simulink model "stable"  (R2020b)
settings: Solver=VariableStepAuto  StartTime=0.0  StopTime=40  RelTol=1e-3
undefined symbols (not defined in the file): c_1, c_2, g, Jp, Jr, L, Lp, Lr, Mp, x0
settings Model: Creator=5470  LastModifiedBy=5470

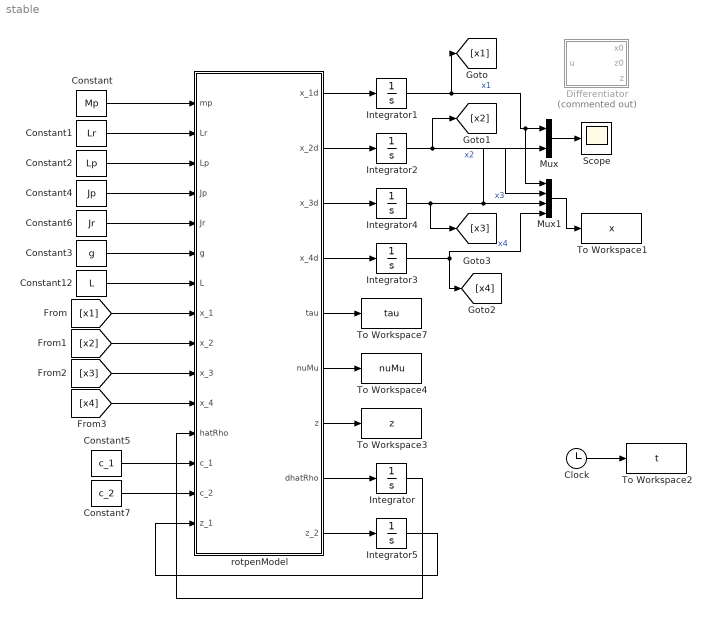
== system stable ==
  Clock : Clock
  Constant : Constant  Value=Mp
  Constant1 : Constant  Value=Lr
  Constant12 : Constant  Value=L
  Constant2 : Constant  Value=Lp
  Constant3 : Constant  Value=g
  Constant4 : Constant  Value=Jp
  Constant5 : Constant  Value=c_1
  Constant6 : Constant  Value=Jr
  Constant7 : Constant  Value=c_2
  Differentiator : Subsystem  Commented=on  TreatAsAtomicUnit=on  mask{n=1, r=3, Ts=-1, filtering=on, nf=1, differentiator_type=Set Homogeneity Degree manually, d=-1, m=1, mu=1}
      mask prompts: n "n ="; r "r ="; Ts "Ts ="; filtering "Enable Filtering"; nf "nf ="; differentiator_type "Type of Differentiator"; d "d ="; m "m ="; mu "mu ="
      mask Callback filtering:
      | zzzzzzzzzz_maskObj = Simulink.Mask.get(gcb);
      | 
      | zzzzzzzzzz_enabled = get_param(gcb, 'filtering');
      | 
      | zzzzzzzzzz_nf_group = zzzzzzzzzz_maskObj.getDialogControl('nf_group');
      | zzzzzzzzzz_nf_group.DialogControls(3).Visible = zzzzzzzzzz_enabled;
      | zzzzzzzzzz_maskVisibilities = get_param(gcb,'maskVisibilities');
      | zzzzzzzzzz_maskVisibilities{5} = zzzzzzzzzz_enabled;
      | set_param(gcb,'maskVisibilities', zzzzzzzzzz_maskVisibilities);
      | if(strcmp(zzzzzzzzzz_enabled, 'off') == 1)
      |     set_param(gcb, 'nf', '0');
      | end
      | 
      | clear zzzzzzzzzz_nf_group zzzzzzzzzz_enabled zzzzzzzzzz_maskVisibilities zzzzzzzzzz_maskObj;
      mask TypeOptions differentiator_type: Linear Differentiator | Robust Exact Differentiator | Uniform Robust Exact Differentiator | Set Homogeneity Degree manually
      mask Callback differentiator_type:
      | zzzzzzzzzz_maskObj = Simulink.Mask.get(gcb);
      | 
      | zzzzzzzzzz_diff_type = get_param(gcb, 'differentiator_type');
      | zzzzzzzzzz_enabled_m = 'on';
      | zzzzzzzzzz_enabled = 'on';
      | zzzzzzzzzz_enabled_m2 = 'off';
      | zzzzzzzzzz_enabled_m3 = 'off';
      | 
      | zzzzzzzzzz_val_m = str2double(get_param(gcb, 'm'));
      | 
      | if(strcmp(zzzzzzzzzz_diff_type, 'Set Homogeneity Degree manually') == 1)
      |     zzzzzzzzzz_enabled_m3 = 'on';
      | else
      |     zzzzzzzzzz_enabled = 'off';
      |     if(strcmp(zzzzzzzzzz_diff_type, 'Linear Differentiator') == 1)
      |         set_param(gcb, 'd', '0');
      |         if(zzzzzzzzzz_val_m == 2)
      |             set_param(gcb, 'm', '1');
      |         end
      |     elseif(strcmp(zzzzzzzzzz_diff_type, 'Robust Exact Differentiator') == 1)
      |         zzzzzzzzzz_enabled_m2 = 'on';
      | 
      |         set_param(gcb, 'd', '-1');
      |     elseif(strcmp(zzzzzzzzzz_diff_type, 'Uniform Robust Exact Differentiator') == 1)
      |         set_param(gcb, 'd', '-1');
      |         set_param(gcb, 'm', '2');
      | 
      |         zzzzzzzzzz_enabled_m = 'off';
      |     end
      | end
      | 
      | zzzzzzzzzz_d_group = zzzzzzzzzz_maskObj.getDialogControl('d_group');
      | zzzzzzzzzz_d_group.DialogControls(2).Visible = zzzzzzzzzz_enabled;
      | zzzzzzzzzz_maskVisibilities = get_param(gcb,'maskVisibilities');
      | zzzzzzzzzz_maskVisibilities{7} = zzzzzzzzzz_enabled;
      | 
      | zzzzzzzzzz_m_group = zzzzzzzzzz_maskObj.getDialogControl('m_group');
      | zzzzzzzzzz_m_group.Visible = zzzzzzzzzz_enabled_m;
      | zzzzzzzzzz_m_group.DialogControls(2).Visible = zzzzzzzzzz_enabled_m2;
      | zzzzzzzzzz_m_group.DialogControls(3).Visible = zzzzzzzzzz_enabled_m3;
      | set_param(gcb,'maskVisibilities', zzzzzzzzzz_maskVisibilities);
      | 
      | clear zzzzzzzzzz_d_group zzzzzzzzzz_maskVisibilities zzzzzzzzzz_m_group zzzzzzzzzz_enabled_m;
      | clear zzzzzzzzzz_enabled_m2 zzzzzzzzzz_enabled_m3 zzzzzzzzzz_enabled zzzzzzzzzz_diff_type;
      | clear zzzzzzzzzz_val_m;
      | 
      | 
      | 
      | zzzzzzzzzz_val_m = str2double(get_param(gcb, 'm'));
      | zzzzzzzzzz_val_d = str2double(get_param(gcb, 'd'));
      | zzzzzzzzzz_enabled_mu = 'off';
      | if((isnan(zzzzzzzzzz_val_m) || zzzzzzzzzz_val_m == 2) && (isnan(zzzzzzzzzz_val_d) || zzzzzzzzzz_val_d == -1))
      |     zzzzzzzzzz_enabled_mu = 'on';
      | end
      | zzzzzzzzzz_maskObj.getDialogControl('mu_group').Visible = zzzzzzzzzz_enabled_mu;
      | clear zzzzzzzzzz_val_m zzzzzzzzzz_val_d zzzzzzzzzz_enabled_mu zzzzzzzzzz_maskObj;
      | clear zzzzzzzzzz_maskObj
      mask Callback d:
      | zzzzzzzzzz_maskObj = Simulink.Mask.get(gcb);
      | zzzzzzzzzz_val_m = str2double(get_param(gcb, 'm'));
      | zzzzzzzzzz_val_d = str2double(get_param(gcb, 'd'));
      | zzzzzzzzzz_enabled_mu = 'off';
      | if((isnan(zzzzzzzzzz_val_m) || zzzzzzzzzz_val_m == 2) && (isnan(zzzzzzzzzz_val_d) || zzzzzzzzzz_val_d == -1))
      |     zzzzzzzzzz_enabled_mu = 'on';
      | end
      | zzzzzzzzzz_maskObj.getDialogControl('mu_group').Visible = zzzzzzzzzz_enabled_mu;
      | clear zzzzzzzzzz_val_m zzzzzzzzzz_val_d zzzzzzzzzz_enabled_mu zzzzzzzzzz_maskObj;
      | clear zzzzzzzzzz_maskObj
      mask Callback m:
      | zzzzzzzzzz_maskObj = Simulink.Mask.get(gcb);
      | zzzzzzzzzz_val_m = str2double(get_param(gcb, 'm'));
      | zzzzzzzzzz_val_d = str2double(get_param(gcb, 'd'));
      | zzzzzzzzzz_enabled_mu = 'off';
      | if((isnan(zzzzzzzzzz_val_m) || zzzzzzzzzz_val_m == 2) && (isnan(zzzzzzzzzz_val_d) || zzzzzzzzzz_val_d == -1))
      |     zzzzzzzzzz_enabled_mu = 'on';
      | end
      | zzzzzzzzzz_maskObj.getDialogControl('mu_group').Visible = zzzzzzzzzz_enabled_mu;
      | clear zzzzzzzzzz_val_m zzzzzzzzzz_val_d zzzzzzzzzz_enabled_mu zzzzzzzzzz_maskObj;
      | clear zzzzzzzzzz_maskObj
      mask DialogControl DescGroupVar Prompt: Differentiator Toolbox v3
      mask DialogControl DescTextVar Prompt: This block provides estimates of the derivatives of the input signal.
      mask DialogControl DescTextVar_2 Prompt: The first scalar output x0 provides a convergence measure. Increase the robustness factor 'r' to ensure that this signal converges to a sufficiently small neighborhood of zero.
      mask DialogControl DescTextVar_3 Prompt: The second output z0 is an estimate of the input signal.
      mask DialogControl DescTextVar_4 Prompt: The third output z is a vector containing the estimated derivatives of the input signal. The length of this vector equals the chosen differentiaton order 'n'.
      mask DialogControl n_group Prompt: Differentiation Order
      mask DialogControl n_desc Prompt: Number of derivatives to be estimated for input signal.
      mask DialogControl r_group Prompt: Robustness Factor
      mask DialogControl r_desc Prompt: Set r to a positive value. This value is proportional to the continuous time closed loop eigenvalues.
      mask DialogControl Ts_group Prompt: Step size
      mask DialogControl Ts_desc Prompt: Simulation Sample Time (-1 for inherited).
      mask DialogControl Advanced Prompt: Advanced Options
      mask DialogControl nf_group Prompt: Filter Options
      mask DialogControl DescTextVar_copy Prompt: Use the filtering option, if there is noise present. Adjust the Filtering Order 'nf' to achieve better estimations for the derivatives. Usually, a filtering order of 1 or 2 is sufficient.
      mask DialogControl nf_desc Prompt: Filtering Order.
      mask DialogControl d_group Prompt: Differentiator Options
      mask DialogControl d_desc Prompt: Set the homogeneity degree to a value between -1 (Robust Exact Differentiator) and 0 (Linear Differentiator).
      mask DialogControl m_group Prompt: Discretization Method
      mask DialogControl m_desc Prompt: Select m out of {0, 1}, where 0 corresponds to Forward Euler eigenvalue mapping and 1 corresponds to Matching Approach.
      mask DialogControl m_desc_copy Prompt: Set m to 2 for Uniform Robust Exact Differentiator behavior.
      mask DialogControl m_desc_copy_copy Prompt: Set m to 2 for Uniform Robust Exact Differentiator behavior (only available for d=-1).
      mask DialogControl mu_group Prompt: Eigenvalue tuning gain for Uniform RED
      mask DialogControl mu_desc Prompt: Set mu to a positive value. mu is a tuning gain for the eigenvalue selection of the Uniform Robust Exact Differentiator.
      mask Display:
      | image('image.png');
      | port_label('input', 1, 'u')
      | port_label('output', 1, 'x0')
      | port_label('output', 2, 'z0')
      | port_label('output', 3, 'z')
  Integrator : Integrator
  Integrator1 : Integrator  InitialCondition=x0(1)
  Integrator2 : Integrator  InitialCondition=x0(2)
  Integrator3 : Integrator  InitialCondition=x0(4)
  Integrator4 : Integrator  InitialCondition=x0(3)
  Integrator5 : Integrator
  Mux : Mux  Inputs=2
  Mux1 : Mux
  Scope : Scope
  To Workspace1 : ToWorkspace  VariableName=x  SampleTime=-1
  To Workspace2 : ToWorkspace  VariableName=t  SampleTime=-1
  To Workspace3 : ToWorkspace  VariableName=z  SampleTime=-1
  To Workspace4 : ToWorkspace  VariableName=nuMu  SampleTime=-1
  To Workspace7 : ToWorkspace  VariableName=tau  SampleTime=-1
  rotpenModel : MATLAB Function  TreatAsAtomicUnit=on
  wires:
  rotpenModel/4(x_4d) -> Integrator3/1
  Integrator2/1 -> Mux1/2, [x2]  "x2"
  Integrator3/1 -> [x4], Mux1/4  "x4"
  rotpenModel/2(x_2d) -> Integrator2/1
  rotpenModel/3(x_3d) -> Integrator4/1
  Integrator4/1 -> [x3], Mux1/3, Mux/2  "x3"
  Mux/1 -> Scope/1
  rotpenModel/5(tau) -> To Workspace7/1
  Integrator/1 -> rotpenModel/12(hatRho)
  Constant12/1 -> rotpenModel/7(L)
  rotpenModel/7(z) -> To Workspace3/1
  Constant2/1 -> rotpenModel/3(Lp)
  Constant5/1 -> rotpenModel/13(c_1)
  Constant3/1 -> rotpenModel/6(g)
  rotpenModel/8(dhatRho) -> Integrator/1
  rotpenModel/6(nuMu) -> To Workspace4/1
  Constant/1 -> rotpenModel/1(mp)
  Constant6/1 -> rotpenModel/5(Jr)
  rotpenModel/1(x_1d) -> Integrator1/1
  Integrator1/1 -> [x1], Mux1/1, Mux/1  "x1"
  Constant1/1 -> rotpenModel/2(Lr)
  Constant4/1 -> rotpenModel/4(Jp)
  Constant7/1 -> rotpenModel/14(c_2)
  rotpenModel/9(z_2) -> Integrator5/1
  Integrator5/1 -> rotpenModel/15(z_1)
  Mux1/1 -> To Workspace1/1
  [x1] -> rotpenModel/8(x_1)
  [x4] -> rotpenModel/11(x_4)
  [x3] -> rotpenModel/10(x_3)
  [x2] -> rotpenModel/9(x_2)
  Clock/1 -> To Workspace2/1

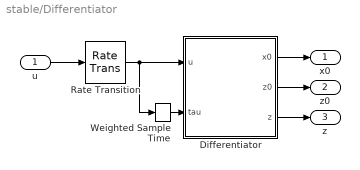
== system stable/Differentiator ==
  u : Inport
  Differentiator : MATLAB Function  TreatAsAtomicUnit=on  SystemSampleTime=Ts
  Rate Transition : RateTransition
  Weighted Sample Time : SampleTimeMath  TsampMathOp=Ts Only
  x0 : Outport  VectorParamsAs1DForOutWhenUnconnected=off
  z0 : Outport  Port=2  VectorParamsAs1DForOutWhenUnconnected=off
  z : Outport  Port=3  VectorParamsAs1DForOutWhenUnconnected=off
  wires:
  Differentiator/3(z) -> z/1
  Differentiator/2(z0) -> z0/1
  Differentiator/1(x0) -> x0/1
  Rate Transition/1 -> Differentiator/1(u), Weighted Sample Time/1
  Weighted Sample Time/1 -> Differentiator/2(tau)
  u/1 -> Rate Transition/1

== matlab function stable/Differentiator/Differentiator ==
  settings: updateMethod=DISCRETE  description=some description
  data: x0 output; z0 output; u input; z output size=n; n parameter; nf parameter; d parameter; r parameter; m parameter; mu parameter; tau input; Ts parameter
function [x0, z0, z] = differentiator(u, n, nf, d, r, m, mu, tau, Ts)
    % Calculates the derivatives up to n-th order of a given signal u
    %   u...  signal vector
    %   n...  maximum order of derivative
    %   nf... filtering order
    %   r...  robustness factor
    %   d...  homogeneity factor: between -1 for Robust Exact Differentiator and 0 for Linear Differentiator
    %   m...  discretization method: 
    %       0 for Forward Euler
    %       1 for Matching Approach
    %       2 for Uniform RED
    %   mu... tuning parameter for Uniform RED eigenvalues
    %   Ts... discretization time
    % 
    % outputs:
    %   x0... error signal (help for tuning r), should converge towards 0
    %   z0... containing the estimated original signal
    %   z ... containing the estimated signal derivatives (n elements)

    persistent Phi bD So_inv_lastCol sys_n zp,

    if isempty(zp)
        CheckParameters(n, nf, d, r, m, mu, Ts, tau);
        
        sys_n = n+nf+1;
        zp = zeros(sys_n,1);

        A = diag(ones(sys_n-1,1),1);

        if(nf > 0)
            b = [zeros(nf-1,1); -1; zeros(n+1,1)];
        else
            b = zeros(n+nf+1,1);
        end

        P = tau*[A, b; zeros(1,sys_n+1)];

        P = expm(P);
        Phi = P(1:sys_n, 1:sys_n);
        bD = P(1:sys_n, sys_n+1);

        U = ((0:sys_n-1)'*ones(1,sys_n));
        U = U.^(ones(sys_n,1)*(0:sys_n-1)) * diag(1./factorial(0:sys_n-1));
        V_inv = diag(1./tau.^(0:sys_n-1));
        So_inv = V_inv / U;
        So_inv_lastCol = So_inv * [zeros(sys_n-1,1);1];
    end
    
    x0 = err(nf, u, zp(1));
    if(m == 2)
        z_eig = disc_eigenvalues_URED(x0, sys_n, r, mu, tau);
    else
        s = cont_eigenvalues(x0, sys_n, d, r);
        z_eig = disc_eigenvalues(m, s, tau);
    end
    
    if(sys_n > 11)
        lambda = ackerman(Phi, sys_n, z_eig, So_inv_lastCol);
    else
        lambda = ackerman_precomputed(sys_n, tau, z_eig);
    end
    
    z0 = zp(nf+1);
    z = zeros(n,1);
    z(1:n) = zp(nf+2:end);
    zp = step(x0, zp, u, Phi, bD, lambda);
end %differentiator

function x0 = err(nf, u, first_state)
    if(nf > 0)
        x0 = -first_state;
    else
        x0 = u - first_state;
    end
end %error

function s = cont_eigenvalues(x0, sys_n, d, r)
    s = -r*(abs(x0)).^(d / (1-d*(sys_n-1)));
end %cont_eigenvalues

function z = disc_eigenvalues(m, s, tau)
    if(m == 0)
        if(isinf(s))
            z = 0;
        else
            z = 1 + tau*s;
        end
    elseif(m == 1)
        z = exp(tau*s);
    else
        z = 0;
    end
end %disc_eigenvalues

function z = disc_eigenvalues_URED(x0, sys_n, r, mu, tau)
    c = abs(x0)^(1.0/sys_n);
    z = c / (tau * r * mu * abs(x0) + c + tau * r);
end %disc_eigenvalues_URED

function lambda = ackerman(Phi, sys_n, z, So_inv_lastCol)
    kappa = (Phi - z*eye(sys_n))^(sys_n);
    lambda = kappa * So_inv_lastCol;
end %ackerman

function lambda = ackerman_precomputed(sys_n, Ts, z)
    z0 = z;
    switch sys_n-1
        case 1
            lambda =  ...
            [
                        2 - z0 - z
             ((z - 1)*(z0 - 1))/Ts
            ];
        case 2
            lambda =  ...
            [
                                       3 - z0 - 2*z
             ((z - 1)*(z + 3*z0 + z*z0 - 5))/(2*Ts)
                         -((z - 1)^2*(z0 - 1))/Ts^2

            ];
        case 3
            lambda =  ...
            [
                                                              4 - z0 - 3*z
             ((z - 1)*(7*z + 11*z0 + 5*z*z0 + 2*z^2*z0 + z^2 - 26))/(6*Ts)
                                       -((z - 1)^2*(2*z0 + z*z0 - 3))/Ts^2
                                                 ((z - 1)^3*(z0 - 1))/Ts^3
            ];
        case 4
            lambda = ...
            [
                                                                                    5 - z0 - 4*z
             ((z - 1)*(23*z + 25*z0 + 13*z*z0 + 7*z^2*z0 + 3*z^3*z0 + 5*z^2 + z^3 - 77))/(12*Ts)
                           -((z - 1)^2*(35*z0 - 2*z + 26*z*z0 + 11*z^2*z0 + z^2 - 71))/(12*Ts^2)
                                                   -((z - 1)^3*(z - 5*z0 - 3*z*z0 + 7))/(2*Ts^3)
                                                                      -((z - 1)^4*(z0 - 1))/Ts^4
            ];
        case 5
            lambda = ...
            [
                                                                                                                 6 - z0 - 5*z
             ((z - 1)*(163*z + 137*z0 + 77*z*z0 + 47*z^2*z0 + 27*z^3*z0 + 12*z^4*z0 + 43*z^2 + 13*z^3 + 3*z^4 - 522))/(60*Ts)
                                   -((z - 1)^2*(45*z0 - 7*z + 40*z*z0 + 25*z^2*z0 + 10*z^3*z0 + 2*z^2 + z^3 - 116))/(12*Ts^2)
                                                          -((z - 1)^3*(8*z - 17*z0 - 16*z*z0 - 7*z^2*z0 + z^2 + 31))/(4*Ts^3)
                                                                                     ((z - 1)^4*(z - 3*z0 - 2*z*z0 + 4))/Ts^4
                                                                                                    ((z - 1)^5*(z0 - 1))/Ts^5
            ];
        case 6
            lambda = ...
            [
                                                                                                                                     7 - z0 - 6*z
             ((z - 1)*(213*z + 147*z0 + 87*z*z0 + 57*z^2*z0 + 37*z^3*z0 + 22*z^4*z0 + 10*z^5*z0 + 63*z^2 + 23*z^3 + 8*z^4 + 2*z^5 - 669))/(60*Ts)
                     -((z - 1)^2*(812*z0 - 232*z + 802*z*z0 + 597*z^2*z0 + 352*z^3*z0 + 137*z^4*z0 + 33*z^2 + 38*z^3 + 13*z^4 - 2552))/(180*Ts^2)
                                                       -((z - 1)^3*(39*z - 49*z0 - 57*z*z0 - 39*z^2*z0 - 15*z^3*z0 + 9*z^2 + z^3 + 111))/(8*Ts^3)
                                                                           ((z - 1)^4*(26*z - 35*z0 - 38*z*z0 - 17*z^2*z0 + 5*z^2 + 59))/(6*Ts^4)
                                                                                                  -((z - 1)^5*(3*z - 7*z0 - 5*z*z0 + 9))/(2*Ts^5)
                                                                                                                       -((z - 1)^6*(z0 - 1))/Ts^6
            ];
        case 7
            lambda = ...
            [
                                                                                                                                                                        8 - z0 - 7*z
             ((z - 1)*(1851*z + 1089*z0 + 669*z*z0 + 459*z^2*z0 + 319*z^3*z0 + 214*z^4*z0 + 130*z^5*z0 + 60*z^6*z0 + 591*z^2 + 241*z^3 + 101*z^4 + 38*z^5 + 10*z^6 - 5772))/(420*Ts)
                                  -((z - 1)^2*(938*z0 - 414*z + 994*z*z0 + 819*z^2*z0 + 574*z^3*z0 + 329*z^4*z0 + 126*z^5*z0 + 16*z^2 + 61*z^3 + 36*z^4 + 11*z^5 - 3490))/(180*Ts^2)
                                                     -((z - 1)^3*(1127*z - 967*z0 - 1277*z*z0 - 1077*z^2*z0 - 647*z^3*z0 - 232*z^4*z0 + 357*z^2 + 77*z^3 + 7*z^4 + 2632))/(120*Ts^3)
                                                                                        ((z - 1)^4*(68*z - 56*z0 - 77*z*z0 - 56*z^2*z0 - 21*z^3*z0 + 23*z^2 + 4*z^3 + 115))/(6*Ts^4)
                                                                                                            -((z - 1)^5*(43*z - 46*z0 - 55*z*z0 - 25*z^2*z0 + 10*z^2 + 73))/(6*Ts^5)
                                                                                                                                          ((z - 1)^6*(2*z - 4*z0 - 3*z*z0 + 5))/Ts^6
                                                                                                                                                           ((z - 1)^7*(z0 - 1))/Ts^7
            ];
        case 8
            lambda = ...
            [
                                                                                                                                                                                                    9 - z0 - 8*z
             ((z - 1)*(4437*z + 2283*z0 + 1443*z*z0 + 1023*z^2*z0 + 743*z^3*z0 + 533*z^4*z0 + 365*z^5*z0 + 225*z^6*z0 + 105*z^7*z0 + 1497*z^2 + 657*z^3 + 307*z^4 + 139*z^5 + 55*z^6 + 15*z^7 - 13827))/(840*Ts)
                -((z - 1)^2*(29531*z0 - 18254*z + 32926*z*z0 + 29013*z^2*z0 + 22468*z^3*z0 + 15293*z^4*z0 + 8622*z^5*z0 + 3267*z^6*z0 - 733*z^2 + 2172*z^3 + 1787*z^4 + 898*z^5 + 261*z^6 - 127251))/(5040*Ts^2)
                                                      -((z - 1)^3*(3777*z - 2403*z0 - 3457*z*z0 - 3302*z^2*z0 - 2442*z^3*z0 - 1367*z^4*z0 - 469*z^5*z0 + 1462*z^2 + 442*z^3 + 87*z^4 + 5*z^5 + 7667))/(240*Ts^3)
                                                                            ((z - 1)^4*(5572*z - 3207*z0 - 5092*z*z0 - 4682*z^2*z0 - 2852*z^3*z0 - 967*z^4*z0 + 2522*z^2 + 772*z^3 + 127*z^4 + 7807))/(240*Ts^4)
                                                                                                                -((z - 1)^5*(122*z - 81*z0 - 125*z*z0 - 95*z^2*z0 - 35*z^3*z0 + 50*z^2 + 10*z^3 + 154))/(6*Ts^5)
                                                                                                                                         ((z - 1)^6*(42*z - 39*z0 - 50*z*z0 - 23*z^2*z0 + 11*z^2 + 59))/(4*Ts^6)
                                                                                                                                                                -((z - 1)^7*(5*z - 9*z0 - 7*z*z0 + 11))/(2*Ts^7)
                                                                                                                                                                                      -((z - 1)^8*(z0 - 1))/Ts^8
            ];
        case 9
            lambda = ...
            [
                                                                                                                                                                                                                                  10 - z0 - 9*z
             ((z - 1)*(15551*z + 7129*z0 + 4609*z*z0 + 3349*z^2*z0 + 2509*z^3*z0 + 1879*z^4*z0 + 1375*z^5*z0 + 955*z^6*z0 + 595*z^7*z0 + 280*z^8*z0 + 5471*z^2 + 2531*z^3 + 1271*z^4 + 641*z^5 + 305*z^6 + 125*z^7 + 35*z^8 - 48610))/(2520*Ts)
                    -((z - 1)^2*(32575*z0 - 26477*z + 37754*z*z0 + 34905*z^2*z0 + 28864*z^3*z0 + 21689*z^4*z0 + 14514*z^5*z0 + 8095*z^6*z0 + 3044*z^7*z0 - 2712*z^2 + 2321*z^3 + 2566*z^4 + 1677*z^5 + 788*z^6 + 223*z^7 - 159826))/(5040*Ts^2)
                                  ((z - 1)^3*(180920*z0 - 363543*z + 276981*z*z0 + 287607*z^2*z0 + 240602*z^3*z0 + 165702*z^4*z0 + 88737*z^5*z0 + 29531*z^6*z0 - 161922*z^2 - 60422*z^3 - 17337*z^4 - 2931*z^5 + 16*z^6 - 663941))/(15120*Ts^3)
                                                                                ((z - 1)^4*(9853*z - 4275*z0 - 7488*z*z0 - 7938*z^2*z0 - 6108*z^3*z0 - 3363*z^4*z0 - 1068*z^5*z0 + 5368*z^2 + 2198*z^3 + 638*z^4 + 101*z^5 + 12082))/(240*Ts^4)
                                                                                                        -((z - 1)^5*(6428*z - 3013*z0 - 5444*z*z0 - 5334*z^2*z0 - 3284*z^3*z0 - 1069*z^4*z0 + 3534*z^2 + 1244*z^3 + 229*z^4 + 6709))/(144*Ts^5)
                                                                                                                                                ((z - 1)^6*(129*z - 75*z0 - 126*z*z0 - 99*z^2*z0 - 36*z^3*z0 + 60*z^2 + 13*z^3 + 134))/(4*Ts^6)
                                                                                                                                                                  -((z - 1)^7*(172*z - 145*z0 - 196*z*z0 - 91*z^2*z0 + 49*z^2 + 211))/(12*Ts^7)
                                                                                                                                                                                                     ((z - 1)^8*(3*z - 5*z0 - 4*z*z0 + 6))/Ts^8
                                                                                                                                                                                                                      ((z - 1)^9*(z0 - 1))/Ts^9
            ];
        case 10
            lambda = ...
            [
                                                                                                                                                                                                                                                                   11 - z0 - 10*z
                        ((z - 1)*(17819*z + 7381*z0 + 4861*z*z0 + 3601*z^2*z0 + 2761*z^3*z0 + 2131*z^4*z0 + 1627*z^5*z0 + 1207*z^6*z0 + 847*z^7*z0 + 532*z^8*z0 + 252*z^9*z0 + 6479*z^2 + 3119*z^3 + 1649*z^4 + 893*z^5 + 473*z^6 + 233*z^7 + 98*z^8 + 28*z^9 - 55991))/(2520*Ts)
             -((z - 1)^2*(177133*z0 - 181196*z + 211686*z*z0 + 202949*z^2*z0 + 175852*z^3*z0 + 140985*z^4*z0 + 104102*z^5*z0 + 68899*z^6*z0 + 38136*z^7*z0 + 14258*z^8*z0 - 27739*z^2 + 10278*z^3 + 16165*z^4 + 12728*z^5 + 7611*z^6 + 3454*z^7 + 962*z^8 - 976263))/(25200*Ts^2)
                                   ((z - 1)^3*(420475*z0 - 1040321*z + 675075*z*z0 + 744585*z^2*z0 + 676405*z^3*z0 + 526605*z^4*z0 + 346845*z^5*z0 + 180175*z^6*z0 + 58635*z^7*z0 - 514467*z^2 - 222035*z^3 - 80075*z^4 - 21303*z^5 - 2669*z^6 + 427*z^7 - 1748357))/(30240*Ts^3)
                                                             ((z - 1)^4*(994506*z - 341693*z0 - 643092*z*z0 - 750990*z^2*z0 - 665660*z^3*z0 - 462765*z^4*z0 - 238632*z^5*z0 - 72368*z^6*z0 + 617430*z^2 + 304040*z^3 + 118155*z^4 + 33126*z^5 + 5084*z^6 + 1102859))/(15120*Ts^4)
                                                                                                           -((z - 1)^5*(24135*z - 8591*z0 - 17305*z*z0 - 19830*z^2*z0 - 15730*z^3*z0 - 8555*z^4*z0 - 2565*z^5*z0 + 16010*z^2 + 7550*z^3 + 2445*z^4 + 427*z^5 + 22009))/(288*Ts^5)
                                                                                                                                      ((z - 1)^6*(18188*z - 7513*z0 - 14948*z*z0 - 15378*z^2*z0 - 9548*z^3*z0 - 3013*z^4*z0 + 11418*z^2 + 4388*z^3 + 853*z^4 + 15553))/(240*Ts^6)
                                                                                                                                                                        -((z - 1)^7*(1139*z - 605*z0 - 1085*z*z0 - 875*z^2*z0 - 315*z^3*z0 + 581*z^2 + 133*z^3 + 1027))/(24*Ts^7)
                                                                                                                                                                                                          ((z - 1)^8*(56*z - 44*z0 - 62*z*z0 - 29*z^2*z0 + 17*z^2 + 62))/(3*Ts^8)
                                                                                                                                                                                                                                -((z - 1)^9*(7*z - 11*z0 - 9*z*z0 + 13))/(2*Ts^9)
                                                                                                                                                                                                                                                     -((z - 1)^10*(z0 - 1))/Ts^10
            ];
        otherwise
            lambda = zeros(sys_n, 1);
    end
end %ackerman_precomputed

function z_new = step(x0, z, u, Phi, bD, lambda)
    z_new = Phi*z + bD * u + lambda*x0;
end %step

function CheckParameters(n, nf, d, r, m, mu, Ts, tau)
    if(isnan(n) || n <= 0),   error('n must be an integer value greater than 0.'), end
    if(isnan(nf) || nf < 0),  error('nf must be an integer value greater than or equal to 0.'), end
    if(isnan(d) || d > 0 || d < -1), error('d must be a value between -1 and 0.'), end
    if(isnan(r) || r < 0),    error('r must be a positive value.'), end
    if(isnan(m) || ~any([0,1,2] == m)), error('m must be out of the set {0,1,2}.'), end
    if(isnan(mu) || mu < 0),  error('mu must be a positive value.'), end
    
    if(isnan(Ts) || (Ts <= 0 && Ts ~= -1)), error('Ts must be a positive value or -1 for inherited step size.'), end
    if(Ts == -1 && tau <= 0)
        error('Inherited step size could not be determined.')
    end
    if(Ts ~= -1 && tau ~= Ts)
        error('Not inherited Ts must equal tau.')
    end
    if(m == 2 && d ~= -1), error('Uniform RED (m = 2) is only allowed with RED (d = -1).'), end
end %CheckParameters

== matlab function stable/rotpenModel ==
  data: x_1d output; x_2d output; x_3d output; x_4d output; tau output; nuMu output; z output; mp input; Lr input; Lp input; Jp input; Jr input; g input; L input; x_1 input; x_2 input; x_3 input; x_4 input; hatRho input; dhatRho output; c_1 input; c_2 input; z_1 input; z_2 output
function [x_1d,x_2d,x_3d,x_4d,tau, nuMu,z,dhatRho,z_2]  = rotpenModel(mp,Lr,Lp,Jp,Jr,g,L,x_1,x_2,x_3,x_4,hatRho,c_1,c_2,z_1)
% 
% x_1=q(1);
% x_3=q(2);
% 
% x_2=dq(1);
% x_4=dq(2);

b_1= Jr + mp*Lr^2 + 0.25*mp*Lp^2;
b_2= 0.25*mp*Lp^2;
b_3= 0.5*mp*Lp*Lr;
b_4= Jp +b_2;
b_5= 0.5*mp*Lp*g;

% % % Quanser Model
% % 
% % states
% % % 
% M=[mp*Lr^2+0.25*mp*Lp^2-0.25*mp*Lp^2*(cos(x_3)^2)+Jr, -0.5*mp*Lp*Lr*cos(x_3);
%    -0.5*mp*Lp*Lr*cos(x_3), Jp+0.25*mp*Lp^2];
% % % Coriolis Forces
% C=[0.5*mp*Lp^2*sin(x_3)*cos(x_3)*x_4, 0.5*mp*Lp*Lr*sin(x_3)*x_4 ;
%    -0.25*mp*Lp^2*cos(x_3)*sin(x_3)*x_2, 0];
% % % Gravity vector
% G=[0 ; -0.5*mp*Lp*g*sin(x_3)];
% % % Input Matrix
% B=[1; 0];
% % Viscous Frictions
fv=[0.0024, 0; 0, 0.0024];
% % 
B_p= 0.0024;
B_r= 0.0024;
% % 
%% Control law

% if (-0.01<cos(x_3)) && (cos(x_3)<0.01)
%     z_1=x_1;
% else
%       z_1=x_1 - (b_4/b_3)*log((sin(x_3)+1)/cos(x_3));
% end
% z_1=x_1 - (b_4/b_3)*log((sin(x_3)+1)/cos(x_3));

z_2=x_2 - (b_4*x_4)/(b_3*cos(x_3));

z_3= tan(x_3);
z_4= (1+tan(x_3)^2)*x_4;

z=[z_1; z_2; z_3; z_4];

%% 4-order 

% Phi = -((b_2/b_3)*(1/sqrt(1 + z_3^2) )*(z_2 + (b_4*z_4/sqrt(1 + z_3^2))/b_3)^2 + b_4*z_4^2/((1 + z_3^2)^(3/2))/b_3 +b_5/b_3)*z_3;
 
% Z = [z_1; z_2 ; z_3 ; z_4];
% K = [0.35; 0.7; 24;	8];
%
%   nu = -K'*z - kappa;
%   nu = -K'*z;

%  nu = -K'*z;
 
%% mu-Mapping
sigma= c_1*z_1 + c_2*z_2;
dsigma= c_1*z_2 - c_2*z_3*(b_5/b_3);

mu_1= z_3-sigma;
mu_2= z_4-dsigma;
% 
% mu=[mu_1; mu_2];
% 
% %% CTA
% 
nuMu=-2.7*L^(2/3)*abs(mu_1)^(1/3)*sign(mu_1) -5.345*L^(1/2)*abs(mu_2)^(1/2)*sign(mu_2) + hatRho;
dhatRho= -1.1*L*sign(mu_1);
% 
nubar=  nuMu-c_1*(b_5/b_3)*z_3 - c_2*(b_5/b_3)*z_4;

%% Feedback Tau
    det=b_4*(b_1-b_2*cos(x_3)^2)-b_3^2*cos(x_3)^2;
    wf=2*b_2*sin(x_3)*cos(x_3)*x_2*x_4+b_3*sin(x_3)*x_4^2;
    nu=(nubar-2*tan(x_3)*(1+tan(x_3)^2)*x_4^2)/(1+tan(x_3)^2);
    f=(b_2*cos(x_3)*sin(x_3)*x_2^2 + b_5*sin(x_3));
    tau= wf+(nu*det-(b_1 - b_2*cos(x_3)^2)*f)/(b_3*cos(x_3));
    w=wf-tau;
    x_1d=x_2;
    x_2d=(b_3*cos(x_3)*f-b_4*w)/det;
    x_3d=x_4;
    x_4d=((b_1-b_2*cos(x_3)^2)*f-b_3*cos(x_3)*w)/det;
